simulink model "kalmanSimulink"  (R2017a)
settings: Solver=FixedStepDiscrete  StartTime=0.0  StopTime=inf  FixedStep=0.001  RelTol=1e-3
libraries: dspsrcs4 x2
settings Model: Creator=Danie  LastModifiedBy=Danie

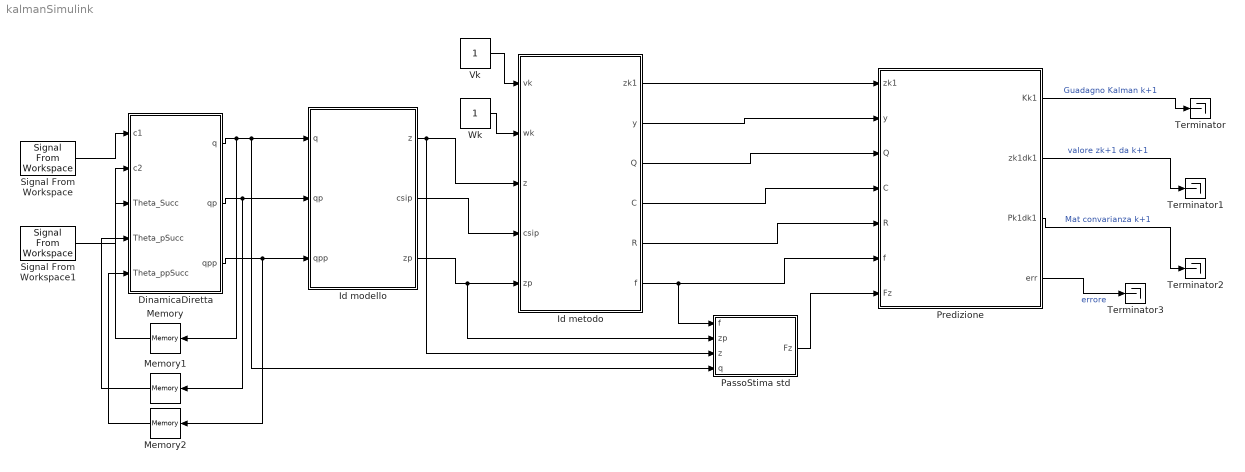
== system kalmanSimulink ==
  DinamicaDiretta : MATLAB Function  TreatAsAtomicUnit=on
  Id metodo : MATLAB Function  TreatAsAtomicUnit=on
  Id modello : MATLAB Function  TreatAsAtomicUnit=on
  Memory : Memory  X0=[0;0]
  Memory1 : Memory  X0=[0;0]
  Memory2 : Memory  X0=[0;0]
  PassoStima std : MATLAB Function  TreatAsAtomicUnit=on
  Predizione : MATLAB Function  TreatAsAtomicUnit=on
  Signal From Workspace : dspsrcs4/Signal From Workspace  X=C1  Ts=0.001  nsamps=1  OutputAfterFinalValue=Setting to zero  ignoreOrWarnInputAndFrameLengths=off  OutputFrames=off
  Signal From Workspace1 : dspsrcs4/Signal From Workspace  X=C2  Ts=0.001  nsamps=1  OutputAfterFinalValue=Setting to zero  ignoreOrWarnInputAndFrameLengths=off  OutputFrames=off
  Terminator{,1..3} (4 alike) : Terminator
  Vk : Constant
  Wk : Constant
  wires:
  Signal From Workspace/1 -> DinamicaDiretta/1(c1)
  Signal From Workspace1/1 -> DinamicaDiretta/2(c2)
  DinamicaDiretta/1(q) -> Memory/1, PassoStima std/4(q), Id modello/1(q)
  DinamicaDiretta/2(qp) -> Memory1/1, Id modello/2(qp)
  DinamicaDiretta/3(qpp) -> Memory2/1, Id modello/3(qpp)
  Id modello/1(z) -> PassoStima std/3(z), Id metodo/3(z)
  Id modello/3(zp) -> PassoStima std/2(zp), Id metodo/5(zp)
  Vk/1 -> Id metodo/1(vk)
  Wk/1 -> Id metodo/2(wk)
  Id metodo/6(f) -> Predizione/6(f), PassoStima std/1(f)
  PassoStima std/1(Fz) -> Predizione/7(Fz)
  Id metodo/2(y) -> Predizione/2(y)
  Id metodo/3(Q) -> Predizione/3(Q)
  Id metodo/4(C) -> Predizione/4(C)
  Id metodo/5(R) -> Predizione/5(R)
  Id metodo/1(zk1) -> Predizione/1(zk1)
  Predizione/1(Kk1) -> Terminator/1  "Guadagno Kalman k+1"
  Predizione/2(zk1dk1) -> Terminator1/1  "valore zk+1 da k+1"
  Predizione/3(Pk1dk1) -> Terminator2/1  "Mat convarianza k+1"
  Id modello/2(csip) -> Id metodo/4(csip)
  Memory/1 -> DinamicaDiretta/3(Theta_Succ)
  Memory1/1 -> DinamicaDiretta/4(Theta_pSucc)
  Memory2/1 -> DinamicaDiretta/5(Theta_ppSucc)
  Predizione/4(err) -> Terminator3/1  "errore"

== matlab function kalmanSimulink/Id modello ==
  data: q input; z output; csip output; qp input; qpp input; zp output
function [z,csip,zp] = IdentificazioneModello(q,qp,qpp)

xp = [qpp ; qp];
csi = ones(2);
z = [qp, q, csi]';
csip = zeros(2); % matrice di zero px1
% p in questi caso = 2
zp = [qpp, qp, csip]';

== matlab function kalmanSimulink/DinamicaDiretta ==
  data: c1 input; q output; c2 input; qp output; qpp output; Theta_Succ input; Theta_pSucc input; Theta_ppSucc input
function [q,qp,qpp]= DinInversa(c1,c2, Theta_Succ, Theta_pSucc, Theta_ppSucc)

tau = [c1;c2];


% Il calcolo della dinamica inversa va fatto passo passo:


Condizioni = [Theta_Succ(1),Theta_Succ(2),Theta_pSucc(1),Theta_pSucc(2)];

[Theta_pSucc, Theta_Succ,Theta_ppSucc] = SoluzioniEquazioniDifferenziali(Condizioni,tau);

 q = Theta_Succ;
 qp = Theta_pSucc;
 qpp = Theta_ppSucc;

== matlab function kalmanSimulink/Id metodo ==
  data: zk1 output; y output; Q output; C output; R output; f output; vk input; wk input; z input; csip input; zp input
function [zk1,y,Q,C,R,f]= IdentificazioneMetodo(vk,wk,z,csip, zp)
dt = 0.001;
f = z + zp*dt;
Vg = [vk 0 ; 0 vk;csip];
zk1 = f+Vg; % z(k+1)
Q = cov(Vg*Vg');
C = [zeros(1,1), eye(1), zeros(1,2)];
y = C*z + wk;
R = cov(wk*wk');

== matlab function kalmanSimulink/PassoStima std ==
  data: f input; Fz output; zp input; z input; q input
function Fz = Stima(f,zp,z, q)
% raccolta dati
theta1pp = zp(1);
theta2pp = zp(2);
theta1p = zp(3);
theta2p = zp(4);
theta1 = q(1);
theta2 = q(2);

zk1M11 = theta1p + theta1pp/1000;
zk1M12 = theta2p + theta2pp/1000;
zk1M21 = theta1 + theta1p/1000;
zk1M22 = theta2 + theta2pp/1000;
% Taylor primo ordine
zk1tMatrix = [ zk1M11, zk1M12; 
               zk1M21, zk1M22;
               1 , 1;
               1 , 1];
           
 Jf1_qp = [1,0;0,1];
 Jf1_q = [0,0;0,0];
%Jf1_qp = jacobian(f(1),z(1));
%Jf1_q = jacobian(f(1),z(2));
Jf1 = [Jf1_qp; Jf1_q];

 Jf2_qp = [1/1000,0;0,1/1000];
 Jf2_q = [1,0;0,1];
%Jf2_qp = jacobian(f(2),z(1));
%Jf2_q = jacobian(f(2),z(2));
Jf2 = [Jf2_qp;  Jf2_q];

Fz = [Jf1, Jf2];

== matlab function kalmanSimulink/Predizione ==
  data: zk1 input; y input; Q input; C input; R input; f input; Fz input; Kk1 output; zk1dk1 output; Pk1dk1 output; err output
function [Kk1,zk1dk1,Pk1dk1,err] = Predizione(zk1,y,Q,C,R,f,Fz)

zk1dk = f;
err = zk1 - zk1dk; % rivedere bene
P = cov(err*err');
Pk1 = Fz*P*Fz'+cov(Q);

Kk1 = Pk1*C'*(C*Pk1*C' +R)^-1;
zk1dk1 = zk1dk+Kk1*(y-C*zk1dk);
Pk1dk1 = Pk1-Kk1*C*Pk1;
